simulink model "Simulink parcial"  (R2021b)
settings: Solver=VariableStepAuto  StartTime=0.0  StopTime=60  RelTol=1e-3
settings Model: Creator=Brayan  LastModifiedBy=Brayan

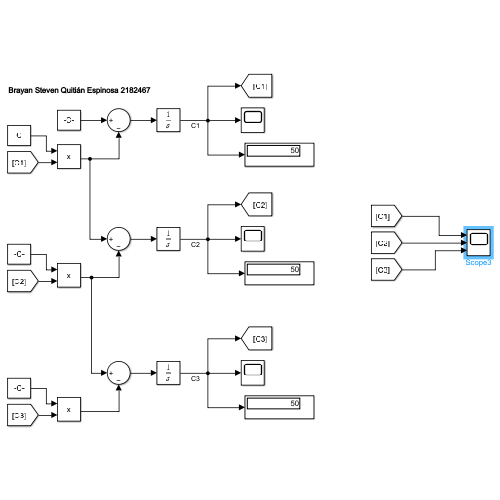
[thumbnail: Simulink's stored preview of the top-level diagram]
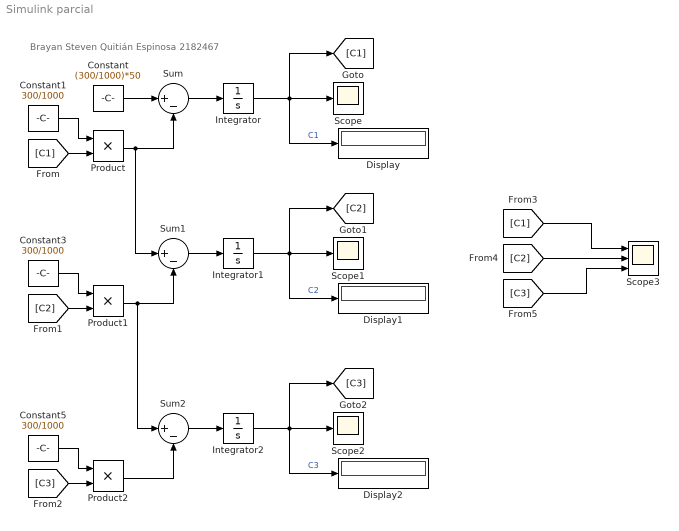
== system Simulink parcial ==
  note: Brayan Steven Quitián Espinosa 2182467
  Constant : Constant  Value=(300/1000)*50
  Constant1 : Constant  Value=300/1000
  Constant3 : Constant  Value=300/1000
  Constant5 : Constant  Value=300/1000
  Display : Display
  Display1 : Display
  Display2 : Display
  Integrator : Integrator  InitialCondition=30
  Integrator1 : Integrator  InitialCondition=30
  Integrator2 : Integrator  InitialCondition=30
  Product : Product
  Product1 : Product
  Product2 : Product
  Scope : Scope
  Scope1 : Scope
  Scope2 : Scope
  Scope3 : Scope  NumInputPorts=3
  Sum : Sum  Inputs=|+-
  Sum1 : Sum  Inputs=|+-
  Sum2 : Sum  Inputs=|+-
  wires:
  Integrator/1 -> Display/1, [C1], Scope/1  "C1"
  Sum/1 -> Integrator/1
  Constant/1 -> Sum/1
  [C1] -> Product/2
  Constant1/1 -> Product/1
  Sum1/1 -> Integrator1/1
  Product/1 -> Sum1/1, Sum/2
  Constant3/1 -> Product1/1
  [C2] -> Product1/2
  Integrator1/1 -> Display1/1, [C2], Scope1/1  "C2"
  Sum2/1 -> Integrator2/1
  Product2/1 -> Sum2/2
  Product1/1 -> Sum2/1, Sum1/2
  Constant5/1 -> Product2/1
  [C3] -> Product2/2
  Integrator2/1 -> Display2/1, [C3], Scope2/1  "C3"
  [C1] -> Scope3/1
  [C2] -> Scope3/2
  [C3] -> Scope3/3
